simulink model "Lab2"  (R2024b)
settings: Solver=FixedStepAuto  StartTime=0.0  StopTime=10.0  RelTol=1e-3  EnableMultiTasking=on
undefined symbols (not defined in the file): BOOL, DINT, OTL, slplc
libraries: simulink x8, arduinolib x3
(part 1 of 8)
settings Model: ExtModeTrigDuration=2  Creator=CoffeElliot  LastModifiedBy=CoffeElliot
settings SolverCC: AutoInsertRateTranBlk=on
settings OptimizationCC: DefaultParameterBehavior=Inlined  EnhancedBackFolding=on  PassReuseOutputArgsAs=Individual arguments  ZeroExternalMemoryAtStartup=off  ZeroInternalMemoryAtStartup=off  MaxStackSize=64  OptimizeBlockOrder=speed  DifferentSizesBufferReuse=on  OptimizationCustomize=off  EfficientTunableParamExpr=on
settings DebuggingCC: ParameterTunabilityLossMsg=error
settings HardwareCC: ProdBitPerInt=16  ProdBitPerPointer=16  ProdBitPerSizeT=16  ProdBitPerPtrDiffT=16  ProdLargestAtomicFloat=None  ProdWordSize=8  ProdHWDeviceType=Atmel->AVR
settings SFSimCC: MATLABDynamicMemAlloc=off
settings RTWCC: Description=Embedded Coder  SystemTargetFile=ert.tlc  HardwareBoard=Arduino Uno  TemplateMakefile=ert_default_tmf  Toolchain=Arduino AVR  BuildConfiguration=Faster Runs
settings CodeAppCC: ForceParamTrailComments=on  IgnoreCustomStorageClasses=off  OperatorAnnotations=on  SimulinkDataObjDesc=on  SFDataObjDesc=on  InsertBlockDesc=on
settings ERTTargetCC: SupportContinuousTime=on  SupportVariableSizeSignals=on  ExtModeTransport=3  ExtModeStaticAlloc=on  ExtModeAutomaticAllocSize=off  ExtModeStaticAllocSize=250  ExtModeMexFile=ext_xcp  ExtModeIntrfLevel=Level2 - Open

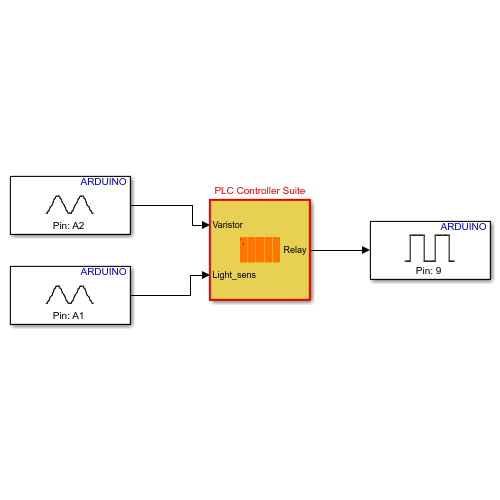
[thumbnail: Simulink's stored preview of the top-level diagram]
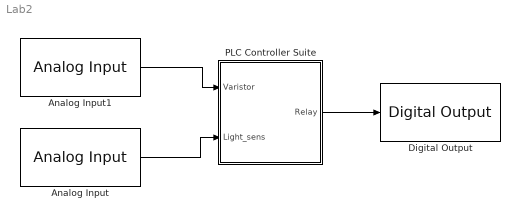
== system Lab2 ==
  Analog Input : arduinolib/Analog Input  pinNumber=1  ReadResultsOnly=off  ConversionTriggerSource=Software  ExternalTriggerType=uint32( 0 )  OutputDataType=uint16  EnableConversionCompleteNotify=off  EnableOuputStatus=off  SampleTime=-1  blockPlatform=arduino
  Analog Input1 : arduinolib/Analog Input  pinNumber=2  ReadResultsOnly=off  ConversionTriggerSource=Software  ExternalTriggerType=uint32( 0 )  OutputDataType=uint16  EnableConversionCompleteNotify=off  EnableOuputStatus=off  SampleTime=-1  blockPlatform=arduino
  Digital Output : arduinolib/Digital Output  pinNumber=9  Direction=output  blockPlatform=arduino
  PLC Controller Suite : Subsystem  TreatAsAtomicUnit=on  mask{PLCBlockType=PLCController, PLCPOUType=PLC Controller}
      mask init:
      | slplc.callbacks.initController(gcb);
      settings: OpenFcn=slplc.callbacks.openPOUBlock(gcb);
      mask Help: web([docroot '/plccoder/ref/plccontrollersuite' '.html']);
      mask DialogControl PLCBlockTitle Prompt: PLC Controller Block
  wires:
  PLC Controller Suite/1(Relay) -> Digital Output/1
  Analog Input1/1 -> PLC Controller Suite/1(Varistor)
  Analog Input/1 -> PLC Controller Suite/2(Light_sens)

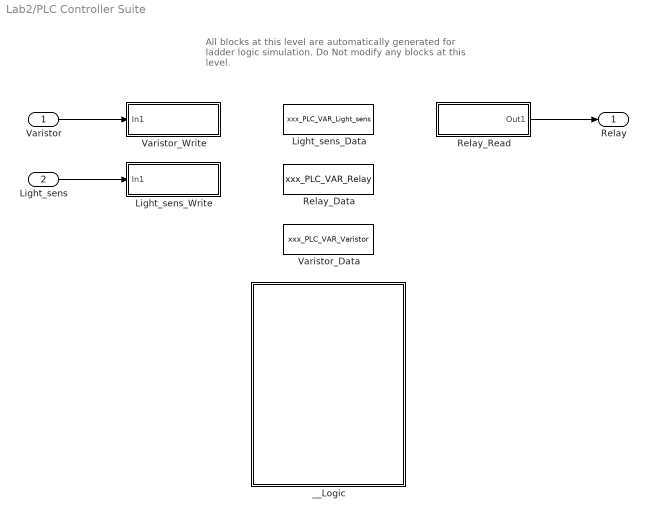
== system Lab2/PLC Controller Suite ==
  note: All blocks at this level are automatically generated for ladder logic simulation.
      | Do Not modify any blocks at this level.
  Varistor : Inport  OutDataTypeStr=double
  Light_sens : Inport  Port=2  OutDataTypeStr=double
  Light_sens_Data : DataStoreMemory  Tag=POUVariable  Priority=10  DataStoreName=xxx_PLC_VAR_Light_sens  InitialValue=1  ShowAdditionalParam=off  OutDataTypeStr=double  Dimensions=1
  Light_sens_Write : Subsystem  Priority=11  DisableCoverage=on  TreatAsAtomicUnit=on  mask{PLCOperandTag=Light_sens, PLCOperandExpression=xxx_PLC_VAR_Light_sens, PLCBlockType=VarWrite, PLCPOUType=VarWrite}
      mask prompts: PLCOperandTag "Operand Tag:"
      mask init:
      | slplc.callbacks.initInstruction(gcb);
      mask Help: web([docroot '/plccoder/ref/varwrite' '.html']);
      mask DialogControl PLCBlockTitle Prompt: Variable Write
      mask Display: disp(get_param(gcb, 'PLCOperandTag'));
  Relay_Data : DataStoreMemory  Tag=POUVariable  Priority=10  DataStoreName=xxx_PLC_VAR_Relay  ShowAdditionalParam=off  OutDataTypeStr=boolean  Dimensions=1
  Relay_Read : Subsystem  Priority=13  DisableCoverage=on  TreatAsAtomicUnit=on  mask{PLCOperandTag=Relay, PLCOperandExpression=xxx_PLC_VAR_Relay, PLCBlockType=VarRead, PLCPOUType=VarRead}
      mask prompts: PLCOperandTag "Operand Tag"
      mask init:
      | block = gcb;
      | maskObj = Simulink.Mask.get(block);
      | maskObj.Display = sprintf('disp(''%s'');', PLCOperandTag);
      | slplc.callbacks.initInstruction(gcb);
      mask Help: web([docroot '/plccoder/ref/varread' '.html']);
      mask DialogControl PLCBlockTitle Prompt: Variable Read
      mask Display: disp('Relay');
  Varistor_Data : DataStoreMemory  Tag=POUVariable  Priority=10  DataStoreName=xxx_PLC_VAR_Varistor  InitialValue=1  ShowAdditionalParam=off  OutDataTypeStr=double  Dimensions=1
  Varistor_Write : Subsystem  Priority=11  DisableCoverage=on  TreatAsAtomicUnit=on  mask{PLCOperandTag=Varistor, PLCOperandExpression=xxx_PLC_VAR_Varistor, PLCBlockType=VarWrite, PLCPOUType=VarWrite}
      mask prompts: PLCOperandTag "Operand Tag:"
      mask init:
      | slplc.callbacks.initInstruction(gcb);
      mask Help: web([docroot '/plccoder/ref/varwrite' '.html']);
      mask DialogControl PLCBlockTitle Prompt: Variable Write
      mask Display: disp(get_param(gcb, 'PLCOperandTag'));
  __Logic : Subsystem  Priority=12  TreatAsAtomicUnit=on
  Relay : Outport
  wires:
  Varistor/1 -> Varistor_Write/1(In1)
  Relay_Read/1(Out1) -> Relay/1
  Light_sens/1 -> Light_sens_Write/1(In1)

== system Lab2/PLC Controller Suite/Light_sens_Write ==
  In1 : Inport
  __CoreVarWrite : Subsystem  Tag=CoreVarWriteBlock  DisableCoverage=on  TreatAsAtomicUnit=on  mask{PLCBlockType=CoreVarWrite}
      mask init:
      | slplc.callbacks.initCoreVariable(gcb, 'write');
      mask DialogControl PLCBlockTitle Prompt: Core Variable Write
  wires:
  In1/1 -> __CoreVarWrite/1(u)

== system Lab2/PLC Controller Suite/Relay_Read ==
  __CoreVarRead : Subsystem  Tag=CoreVarReadBlock  DisableCoverage=on  TreatAsAtomicUnit=on  mask{PLCBlockType=CoreVarRead}
      mask init:
      | slplc.callbacks.initCoreVariable(gcb, 'read');
      mask DialogControl PLCBlockTitle Prompt: Core Variable Read
  Out1 : Outport  VectorParamsAs1DForOutWhenUnconnected=off
  wires:
  __CoreVarRead/1(y) -> Out1/1

== system Lab2/PLC Controller Suite/Varistor_Write ==
  In1 : Inport
  __CoreVarWrite : Subsystem  Tag=CoreVarWriteBlock  DisableCoverage=on  TreatAsAtomicUnit=on  mask{PLCBlockType=CoreVarWrite}
      mask init:
      | slplc.callbacks.initCoreVariable(gcb, 'write');
      mask DialogControl PLCBlockTitle Prompt: Core Variable Write
  wires:
  In1/1 -> __CoreVarWrite/1(u)

== system Lab2/PLC Controller Suite/__Logic ==
  Controller Tags : Subsystem  Tag=ControllerVariableSS  DisableCoverage=on  TreatAsAtomicUnit=on  mask{PLCVarVaristorName=Varistor, PLCVarVaristorAddress=<empty>, PLCVarVaristorMapping=Input Symbol, PLCVarVaristorPortIndex=1, PLCVarVaristorDataType=double, PLCVarVaristorSize=1, PLCVarVaristorInitialValue=1, PLCVarVaristorToDelete=off, PLCVarLight_sensName=Light_sens, PLCVarLight_sensAddress=<empty>, PLCVarLight_sensMapping=Input Symbol, PLCVarLight_sensPortIndex=2, PLCVarLight_sensDataType=double, PLCVarLight_sensSize=1, PLCVarLight_sensInitialValue=1, PLCVarLight_sensToDelete=off, PLCVarRelayName=Relay, PLCVarRelayAddress=<empty>, PLCVarRelayMapping=Output Symbol, PLCVarRelayPortIndex=1, PLCVarRelayDataType=boolean, PLCVarRelaySize=1, PLCVarRelayInitialValue=0, PLCVarRelayToDelete=off}
      mask init:
      | slplc.callbacks.initControllerVarSS(gcb);
      settings: OpenFcn=slplc.callbacks.openControllerVariableSS(gcb);
      mask Help: web([docroot '/plccoder/ref/controllertags' '.html']);
      mask TypeOptions PLCVarVaristorMapping: Global Variable | Input Symbol | Output Symbol
      mask TypeOptions PLCVarVaristorPortIndex: 1 | 2 | 3
      mask TypeOptions PLCVarLight_sensMapping: Global Variable | Input Symbol | Output Symbol
      mask TypeOptions PLCVarLight_sensPortIndex: 1 | 2 | 3
      mask TypeOptions PLCVarRelayMapping: Global Variable | Input Symbol | Output Symbol
      mask TypeOptions PLCVarRelayPortIndex: 1 | 2 | 3
      mask DialogControl PLCBlockTitle Prompt: Global Variable and Symbol Spreadsheet
      mask DialogControl PLCVarListHeaderName Prompt: Name
      mask DialogControl PLCVarListHeaderAddress Prompt: Address (At)
      mask DialogControl PLCVarListHeaderMapping Prompt: Mapping Type
      mask DialogControl PLCVarListHeaderPortIndex Prompt: Port
      mask DialogControl PLCVarListHeaderDataType Prompt: Data Type
      mask DialogControl PLCVarListHeaderSize Prompt: Size
      mask DialogControl PLCVarListHeaderInitialValue Prompt: Initial Value
      mask DialogControl PLCVarListHeaderToDelete Prompt: Delete
  Task : Subsystem  TreatAsAtomicUnit=on  mask{PLCBlockType=Task, PLCPOUType=Task, PLCTaskWatchDog=0}
      settings: OpenFcn=slplc.callbacks.openTaskBlock(gcb);
      mask Help: web([docroot '/plccoder/ref/task' '.html']);
      mask DialogControl PLCBlockTitle Prompt: Task
  Up to Parent POU : Subsystem  DisableCoverage=on  TreatAsAtomicUnit=on  mask{PLCBlockType=OpenParentPOU}
      settings: OpenFcn=slplc.callbacks.openParentPOUBlock(gcb);
      mask Help: web([docroot '/plccoder/ref/uptoparentpou' '.html']);
      mask DialogControl PLCBlockTitle Prompt: Add Single Rung

== system Lab2/PLC Controller Suite/Light_sens_Write/__CoreVarWrite ==
  u : Inport
  DataWrite : DataStoreWrite  DataStoreName=xxx_PLC_VAR_Light_sens  IndexOptions=Index vector (dialog)  Indices=1  OutputSizes=1
  wires:
  u/1 -> DataWrite/1

== system Lab2/PLC Controller Suite/Relay_Read/__CoreVarRead ==
  DataRead : DataStoreRead  DataStoreName=xxx_PLC_VAR_Relay  IndexOptions=Index vector (dialog)  Indices=1  OutputSizes=1
  y : Outport  VectorParamsAs1DForOutWhenUnconnected=off
  wires:
  DataRead/1 -> y/1

== system Lab2/PLC Controller Suite/Varistor_Write/__CoreVarWrite ==
  u : Inport
  DataWrite : DataStoreWrite  DataStoreName=xxx_PLC_VAR_Varistor  IndexOptions=Index vector (dialog)  Indices=1  OutputSizes=1
  wires:
  u/1 -> DataWrite/1

== system Lab2/PLC Controller Suite/__Logic/Controller Tags ==

== system Lab2/PLC Controller Suite/__Logic/Task ==
  Program : Subsystem  TreatAsAtomicUnit=on  mask{PLCPOUType=Program, PLCPOULanguage=LD, PLCBlockType=LDProgram}
      mask prompts: PLCPOUType "POU Type:"
      mask init:
      | slplc.callbacks.initProgram(gcb);
      settings: OpenFcn=slplc.callbacks.openPOUBlock(gcb);
      mask Help: web([docroot '/plccoder/ref/ldprogram' '.html']);
      mask DialogControl PLCBlockTitle Prompt: Program
      mask DialogControl PLCEditPOU Prompt: Edit POU
      mask DialogControl PLCEditInterface Prompt: Edit Variables
  Up to Parent POU : Subsystem  DisableCoverage=on  TreatAsAtomicUnit=on  mask{PLCBlockType=OpenParentPOU}
      settings: OpenFcn=slplc.callbacks.openParentPOUBlock(gcb);
      mask Help: web([docroot '/plccoder/ref/uptoparentpou' '.html']);
      mask DialogControl PLCBlockTitle Prompt: Add Single Rung

== system Lab2/PLC Controller Suite/__Logic/Up to Parent POU ==

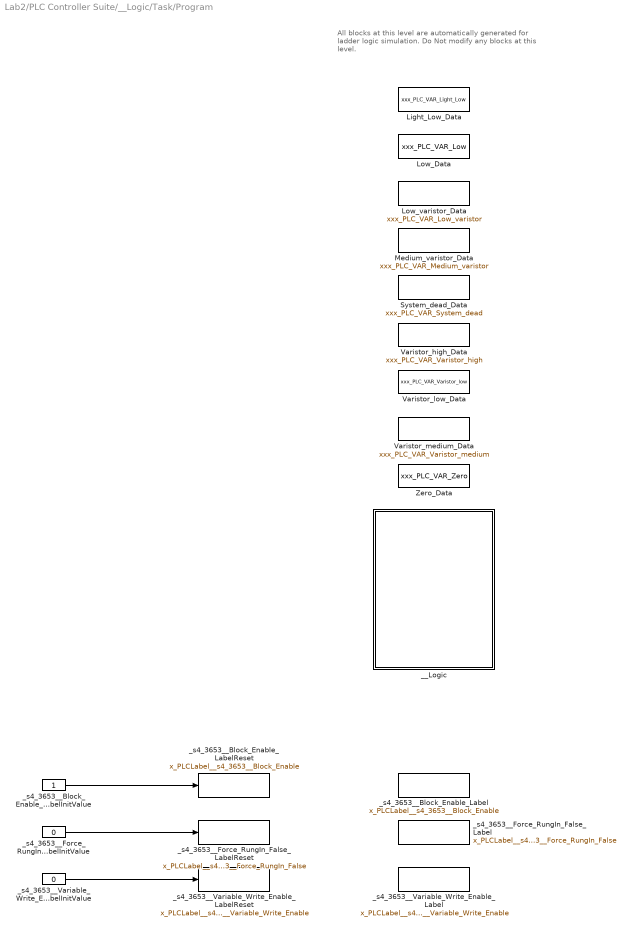
== system Lab2/PLC Controller Suite/__Logic/Task/Program ==
  note: All blocks at this level are automatically generated for ladder logic simulation.
      | Do Not modify any blocks at this level.
  Light_Low_Data : DataStoreMemory  Tag=POUVariable  Priority=10  DataStoreName=xxx_PLC_VAR_Light_Low  InitialValue=false  ShowAdditionalParam=off  OutDataTypeStr=BOOL  Dimensions=1
  Low_Data : DataStoreMemory  Tag=POUVariable  Priority=10  DataStoreName=xxx_PLC_VAR_Low  InitialValue=1000  ShowAdditionalParam=off  OutDataTypeStr=double  Dimensions=1
  Low_varistor_Data : DataStoreMemory  Tag=POUVariable  Priority=10  DataStoreName=xxx_PLC_VAR_Low_varistor  InitialValue=1000  ShowAdditionalParam=off  OutDataTypeStr=double  Dimensions=1
  Medium_varistor_Data : DataStoreMemory  Tag=POUVariable  Priority=10  DataStoreName=xxx_PLC_VAR_Medium_varistor  InitialValue=2500  ShowAdditionalParam=off  OutDataTypeStr=double  Dimensions=1
  System_dead_Data : DataStoreMemory  Tag=POUVariable  Priority=10  DataStoreName=xxx_PLC_VAR_System_dead  InitialValue=false  ShowAdditionalParam=off  OutDataTypeStr=BOOL  Dimensions=1
  Varistor_high_Data : DataStoreMemory  Tag=POUVariable  Priority=10  DataStoreName=xxx_PLC_VAR_Varistor_high  InitialValue=false  ShowAdditionalParam=off  OutDataTypeStr=BOOL  Dimensions=1
  Varistor_low_Data : DataStoreMemory  Tag=POUVariable  Priority=10  DataStoreName=xxx_PLC_VAR_Varistor_low  InitialValue=false  ShowAdditionalParam=off  OutDataTypeStr=BOOL  Dimensions=1
  Varistor_medium_Data : DataStoreMemory  Tag=POUVariable  Priority=10  DataStoreName=xxx_PLC_VAR_Varistor_medium  InitialValue=false  ShowAdditionalParam=off  OutDataTypeStr=BOOL  Dimensions=1
  Zero_Data : DataStoreMemory  Tag=POUVariable  Priority=10  DataStoreName=xxx_PLC_VAR_Zero  InitialValue=10  ShowAdditionalParam=off  OutDataTypeStr=double  Dimensions=1
  __Logic : Subsystem  Priority=12  TreatAsAtomicUnit=on
  _s4_3653__Block_Enable_Label : DataStoreMemory  Priority=10  DataStoreName=x_PLCLabel__s4_3653__Block_Enable  InitialValue=1  ShowAdditionalParam=off  OutDataTypeStr=BOOL  Dimensions=1
  _s4_3653__Block_Enable_LabelInitValue : Constant  OutDataTypeStr=BOOL
  _s4_3653__Block_Enable_LabelReset : DataStoreWrite  Priority=11  DataStoreName=x_PLCLabel__s4_3653__Block_Enable  IndexOptions=Index vector (dialog)  Indices=1  OutputSizes=1
  _s4_3653__Force_RungIn_False_Label : DataStoreMemory  Priority=10  DataStoreName=x_PLCLabel__s4_3653__Force_RungIn_False  ShowAdditionalParam=off  OutDataTypeStr=BOOL  Dimensions=1
  _s4_3653__Force_RungIn_False_LabelInitValue : Constant  Value=0  OutDataTypeStr=BOOL
  _s4_3653__Force_RungIn_False_LabelReset : DataStoreWrite  Priority=11  DataStoreName=x_PLCLabel__s4_3653__Force_RungIn_False  IndexOptions=Index vector (dialog)  Indices=1  OutputSizes=1
  _s4_3653__Variable_Write_Enable_Label : DataStoreMemory  Priority=10  DataStoreName=x_PLCLabel__s4_3653__Variable_Write_Enable  ShowAdditionalParam=off  OutDataTypeStr=BOOL  Dimensions=1
  _s4_3653__Variable_Write_Enable_LabelInitValue : Constant  Value=0  OutDataTypeStr=BOOL
  _s4_3653__Variable_Write_Enable_LabelReset : DataStoreWrite  Priority=11  DataStoreName=x_PLCLabel__s4_3653__Variable_Write_Enable  IndexOptions=Index vector (dialog)  Indices=1  OutputSizes=1
  wires:
  _s4_3653__Block_Enable_LabelInitValue/1 -> _s4_3653__Block_Enable_LabelReset/1
  _s4_3653__Variable_Write_Enable_LabelInitValue/1 -> _s4_3653__Variable_Write_Enable_LabelReset/1
  _s4_3653__Force_RungIn_False_LabelInitValue/1 -> _s4_3653__Force_RungIn_False_LabelReset/1

== system Lab2/PLC Controller Suite/__Logic/Task/Up to Parent POU ==

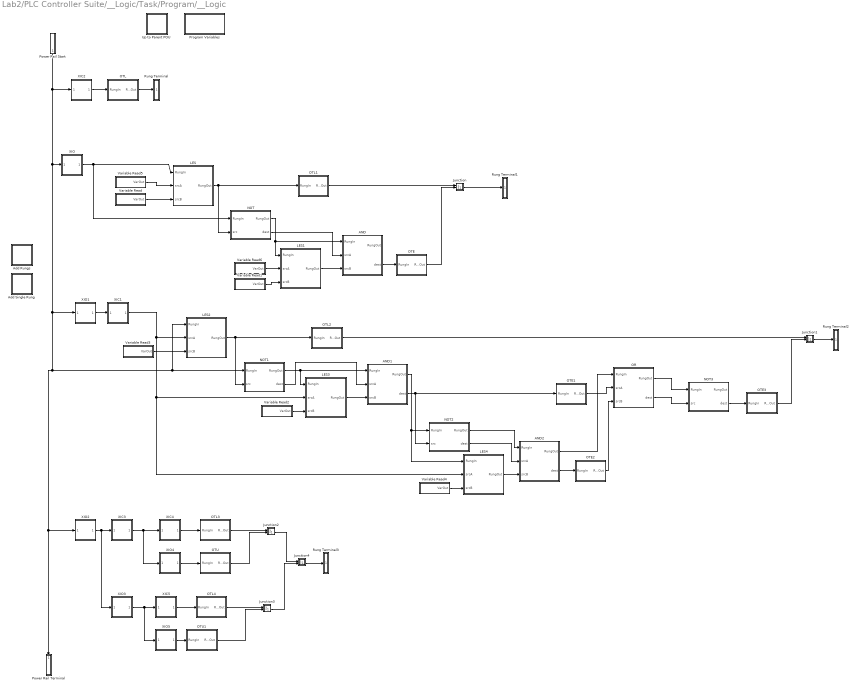
== system Lab2/PLC Controller Suite/__Logic/Task/Program/__Logic ==
  AND : Subsystem  Priority=1  TreatAsAtomicUnit=on  mask{PLCBlockType=AND, PLCPOUType=stdFC}
      mask Help: web([docroot '/plccoder/ref/and' '.html']);
      mask DialogControl PLCBlockTitle Prompt: Bitwise And (AND)
      mask DialogControl PLCBlockDesc Prompt: Perform a bitwise AND operation using the bits in Source A and Source B and place the result in Destination.
      mask Display: disp('AND');
  AND1 : Subsystem  Priority=1  TreatAsAtomicUnit=on  mask{PLCBlockType=AND, PLCPOUType=stdFC}
      mask Help: web([docroot '/plccoder/ref/and' '.html']);
      mask DialogControl PLCBlockTitle Prompt: Bitwise And (AND)
      mask DialogControl PLCBlockDesc Prompt: Perform a bitwise AND operation using the bits in Source A and Source B and place the result in Destination.
      mask Display: disp('AND');
  AND2 : Subsystem  Priority=1  TreatAsAtomicUnit=on  mask{PLCBlockType=AND, PLCPOUType=stdFC}
      mask Help: web([docroot '/plccoder/ref/and' '.html']);
      mask DialogControl PLCBlockTitle Prompt: Bitwise And (AND)
      mask DialogControl PLCBlockDesc Prompt: Perform a bitwise AND operation using the bits in Source A and Source B and place the result in Destination.
      mask Display: disp('AND');
  Add Rungs : Subsystem  DisableCoverage=on  TreatAsAtomicUnit=on  mask{PLCRungNumberToAdd=2, PLCBlockType=AddRungs}
      mask prompts: PLCRungNumberToAdd "Rung Number:"
      mask Help: web([docroot '/plccoder/ref/addrungs' '.html']);
      mask DialogControl PLCAddRungs Prompt: Add Rungs
      mask DialogControl PLCRungAddButton Prompt: Add
      mask DialogControl PLCRungAddButton Callback: slplc.callbacks.addLadderRungs(gcb);
      mask Display: disp(sprintf(['Add' newline 'Rungs']));
  Add Single Rung : Subsystem  DisableCoverage=on  TreatAsAtomicUnit=on  mask{PLCRungNumberToAdd=1, PLCBlockType=AddSingleRung}
      settings: OpenFcn=slplc.callbacks.addLadderRungs(gcb);
      mask Help: web([docroot '/plccoder/ref/addsinglerung' '.html']);
      mask DialogControl PLCAddRung Prompt: Add Single Rung
      mask Display: disp(sprintf(['Add' newline '1 Rung']));
  Junction : Subsystem  DisableCoverage=on  TreatAsAtomicUnit=on  mask{PLCBlockType=Junction, PLCPOUType=BranchJunction}
      mask Help: web([docroot '/plccoder/ref/junction' '.html']);
      mask DialogControl PLCBlockTitle Prompt: Rung Merge Point
      mask DialogControl PLCBlockDesc Prompt: This is the ladder diagram rung merge point.
  Junction1 : Subsystem  DisableCoverage=on  TreatAsAtomicUnit=on  mask{PLCBlockType=Junction, PLCPOUType=BranchJunction}
      mask Help: web([docroot '/plccoder/ref/junction' '.html']);
      mask DialogControl PLCBlockTitle Prompt: Rung Merge Point
      mask DialogControl PLCBlockDesc Prompt: This is the ladder diagram rung merge point.
  Junction2 : Subsystem  DisableCoverage=on  TreatAsAtomicUnit=on  mask{PLCBlockType=Junction, PLCPOUType=BranchJunction}
      mask Help: web([docroot '/plccoder/ref/junction' '.html']);
      mask DialogControl PLCBlockTitle Prompt: Rung Merge Point
      mask DialogControl PLCBlockDesc Prompt: This is the ladder diagram rung merge point.
  Junction3 : Subsystem  DisableCoverage=on  TreatAsAtomicUnit=on  mask{PLCBlockType=Junction, PLCPOUType=BranchJunction}
      mask Help: web([docroot '/plccoder/ref/junction' '.html']);
      mask DialogControl PLCBlockTitle Prompt: Rung Merge Point
      mask DialogControl PLCBlockDesc Prompt: This is the ladder diagram rung merge point.
  Junction4 : Subsystem  DisableCoverage=on  TreatAsAtomicUnit=on  mask{PLCBlockType=Junction, PLCPOUType=BranchJunction}
      mask Help: web([docroot '/plccoder/ref/junction' '.html']);
      mask DialogControl PLCBlockTitle Prompt: Rung Merge Point
      mask DialogControl PLCBlockDesc Prompt: This is the ladder diagram rung merge point.
  LES : Subsystem  Priority=8  TreatAsAtomicUnit=on  mask{PLCBlockType=LES, PLCPOUType=stdFC}
      mask Help: web([docroot '/plccoder/ref/les' '.html']);
      mask DialogControl PLCBlockTitle Prompt: Less Than (LES)
      mask DialogControl PLCBlockDesc Prompt: Test whether Source A is less than Source B.
      mask Display: disp('LES');
  LES1 : Subsystem  Priority=1  TreatAsAtomicUnit=on  mask{PLCBlockType=LES, PLCPOUType=stdFC}
      mask Help: web([docroot '/plccoder/ref/les' '.html']);
      mask DialogControl PLCBlockTitle Prompt: Less Than (LES)
      mask DialogControl PLCBlockDesc Prompt: Test whether Source A is less than Source B.
      mask Display: disp('LES');
  LES2 : Subsystem  Priority=1  TreatAsAtomicUnit=on  mask{PLCBlockType=LES, PLCPOUType=stdFC}
      mask Help: web([docroot '/plccoder/ref/les' '.html']);
      mask DialogControl PLCBlockTitle Prompt: Less Than (LES)
      mask DialogControl PLCBlockDesc Prompt: Test whether Source A is less than Source B.
      mask Display: disp('LES');
  LES3 : Subsystem  Priority=1  TreatAsAtomicUnit=on  mask{PLCBlockType=LES, PLCPOUType=stdFC}
      mask Help: web([docroot '/plccoder/ref/les' '.html']);
      mask DialogControl PLCBlockTitle Prompt: Less Than (LES)
      mask DialogControl PLCBlockDesc Prompt: Test whether Source A is less than Source B.
      mask Display: disp('LES');
  LES4 : Subsystem  Priority=1  TreatAsAtomicUnit=on  mask{PLCBlockType=LES, PLCPOUType=stdFC}
      mask Help: web([docroot '/plccoder/ref/les' '.html']);
      mask DialogControl PLCBlockTitle Prompt: Less Than (LES)
      mask DialogControl PLCBlockDesc Prompt: Test whether Source A is less than Source B.
      mask Display: disp('LES');
  NOT : Subsystem  Priority=1  TreatAsAtomicUnit=on  mask{PLCBlockType=NOT, PLCPOUType=stdFC}
      mask Help: web([docroot '/plccoder/ref/not' '.html']);
      mask DialogControl PLCBlockTitle Prompt: Bitwise Not (NOT)
      mask DialogControl PLCBlockDesc Prompt: Perform a bitwise inversion of the Source and place the result in Destination.
      mask Display: disp('NOT');
  NOT1 : Subsystem  Priority=1  TreatAsAtomicUnit=on  mask{PLCBlockType=NOT, PLCPOUType=stdFC}
      mask Help: web([docroot '/plccoder/ref/not' '.html']);
      mask DialogControl PLCBlockTitle Prompt: Bitwise Not (NOT)
      mask DialogControl PLCBlockDesc Prompt: Perform a bitwise inversion of the Source and place the result in Destination.
      mask Display: disp('NOT');
  NOT2 : Subsystem  Priority=1  TreatAsAtomicUnit=on  mask{PLCBlockType=NOT, PLCPOUType=stdFC}
      mask Help: web([docroot '/plccoder/ref/not' '.html']);
      mask DialogControl PLCBlockTitle Prompt: Bitwise Not (NOT)
      mask DialogControl PLCBlockDesc Prompt: Perform a bitwise inversion of the Source and place the result in Destination.
      mask Display: disp('NOT');
  NOT3 : Subsystem  Priority=1  TreatAsAtomicUnit=on  mask{PLCBlockType=NOT, PLCPOUType=stdFC}
      mask Help: web([docroot '/plccoder/ref/not' '.html']);
      mask DialogControl PLCBlockTitle Prompt: Bitwise Not (NOT)
      mask DialogControl PLCBlockDesc Prompt: Perform a bitwise inversion of the Source and place the result in Destination.
      mask Display: disp('NOT');
  OR : Subsystem  Priority=1  TreatAsAtomicUnit=on  mask{PLCBlockType=OR, PLCPOUType=stdFC}
      mask Help: web([docroot '/plccoder/ref/or' '.html']);
      mask DialogControl PLCBlockTitle Prompt: Bitwise Or
      mask DialogControl PLCBlockDesc Prompt: Perform a bitwise OR operation using the bits in Source A and Source B and place the result in Destination.
      mask Display: disp('OR');
  OTE : Subsystem  Priority=3  TreatAsAtomicUnit=on  mask{PLCOperandTag=Light_Low, PLCBlockType=OTE, PLCPOUType=Coil, PLCOperandExpression=xxx_PLC_VAR_Light_Low}
      mask prompts: PLCOperandTag "Operand Tag:"
      mask init:
      | slplc.callbacks.initInstruction(gcb);
      settings: AttributesFormatString=%<PLCOperandTag>
      mask Help: web([docroot '/plccoder/ref/ote' '.html']);
      mask DialogControl PLCBlockTitle Prompt: Output Energize (OTE)
  OTE1 : Subsystem  Priority=3  TreatAsAtomicUnit=on  mask{PLCOperandTag=Varistor_low, PLCBlockType=OTE, PLCPOUType=Coil, PLCOperandExpression=xxx_PLC_VAR_Varistor_low}
      mask prompts: PLCOperandTag "Operand Tag:"
      mask init:
      | slplc.callbacks.initInstruction(gcb);
      settings: AttributesFormatString=%<PLCOperandTag>
      mask Help: web([docroot '/plccoder/ref/ote' '.html']);
      mask DialogControl PLCBlockTitle Prompt: Output Energize (OTE)
  OTE2 : Subsystem  Priority=3  TreatAsAtomicUnit=on  mask{PLCOperandTag=Varistor_medium, PLCBlockType=OTE, PLCPOUType=Coil, PLCOperandExpression=xxx_PLC_VAR_Varistor_medium}
      mask prompts: PLCOperandTag "Operand Tag:"
      mask init:
      | slplc.callbacks.initInstruction(gcb);
      settings: AttributesFormatString=%<PLCOperandTag>
      mask Help: web([docroot '/plccoder/ref/ote' '.html']);
      mask DialogControl PLCBlockTitle Prompt: Output Energize (OTE)
  OTE3 : Subsystem  Priority=3  TreatAsAtomicUnit=on  mask{PLCOperandTag=Varistor_high, PLCBlockType=OTE, PLCPOUType=Coil, PLCOperandExpression=xxx_PLC_VAR_Varistor_high}
      mask prompts: PLCOperandTag "Operand Tag:"
      mask init:
      | slplc.callbacks.initInstruction(gcb);
      settings: AttributesFormatString=%<PLCOperandTag>
      mask Help: web([docroot '/plccoder/ref/ote' '.html']);
      mask DialogControl PLCBlockTitle Prompt: Output Energize (OTE)
  OTL : Subsystem  Priority=3  TreatAsAtomicUnit=on  mask{PLCOperandTag=Relay, PLCBlockType=OTL, PLCPOUType=Coil, PLCOperandExpression=xxx_PLC_VAR_Relay}
      mask prompts: PLCOperandTag "Operand Tag:"
      mask init:
      | slplc.callbacks.initInstruction(gcb);
      settings: AttributesFormatString=%<PLCOperandTag>
      mask Help: web([docroot '/plccoder/ref/otl' '.html']);
      mask DialogControl PLCBlockTitle Prompt: Output Latch (OTL)
      mask Display: disp('L');
  OTL1 : Subsystem  Priority=9  TreatAsAtomicUnit=on  mask{PLCOperandTag=System_dead, PLCBlockType=OTL, PLCPOUType=Coil, PLCOperandExpression=xxx_PLC_VAR_System_dead}
      mask prompts: PLCOperandTag "Operand Tag:"
      mask init:
      | slplc.callbacks.initInstruction(gcb);
      settings: AttributesFormatString=%<PLCOperandTag>
      mask Help: web([docroot '/plccoder/ref/otl' '.html']);
      mask DialogControl PLCBlockTitle Prompt: Output Latch (OTL)
      mask Display: disp('L');
  OTL2 : Subsystem  Priority=3  TreatAsAtomicUnit=on  mask{PLCOperandTag=Relay, PLCBlockType=OTL, PLCPOUType=Coil, PLCOperandExpression=xxx_PLC_VAR_Relay}
      mask prompts: PLCOperandTag "Operand Tag:"
      mask init:
      | slplc.callbacks.initInstruction(gcb);
      settings: AttributesFormatString=%<PLCOperandTag>
      mask Help: web([docroot '/plccoder/ref/otl' '.html']);
      mask DialogControl PLCBlockTitle Prompt: Output Latch (OTL)
      mask Display: disp('L');
  OTL3 : Subsystem  Priority=3  TreatAsAtomicUnit=on  mask{PLCOperandTag=System_dead, PLCBlockType=OTL, PLCPOUType=Coil, PLCOperandExpression=xxx_PLC_VAR_System_dead}
      mask prompts: PLCOperandTag "Operand Tag:"
      mask init:
      | slplc.callbacks.initInstruction(gcb);
      settings: AttributesFormatString=%<PLCOperandTag>
      mask Help: web([docroot '/plccoder/ref/otl' '.html']);
      mask DialogControl PLCBlockTitle Prompt: Output Latch (OTL)
      mask Display: disp('L');
  OTL4 : Subsystem  Priority=3  TreatAsAtomicUnit=on  mask{PLCOperandTag=Relay, PLCBlockType=OTL, PLCPOUType=Coil, PLCOperandExpression=xxx_PLC_VAR_Relay}
      mask prompts: PLCOperandTag "Operand Tag:"
      mask init:
      | slplc.callbacks.initInstruction(gcb);
      settings: AttributesFormatString=%<PLCOperandTag>
      mask Help: web([docroot '/plccoder/ref/otl' '.html']);
      mask DialogControl PLCBlockTitle Prompt: Output Latch (OTL)
      mask Display: disp('L');
  OTU : Subsystem  Priority=4  TreatAsAtomicUnit=on  mask{PLCOperandTag=Relay, PLCBlockType=OTU, PLCPOUType=Coil, PLCOperandExpression=xxx_PLC_VAR_Relay}
      mask prompts: PLCOperandTag "Operand Tag:"
      mask init:
      | slplc.callbacks.initInstruction(gcb);
      settings: AttributesFormatString=%<PLCOperandTag>
      mask Help: web([docroot '/plccoder/ref/otu' '.html']);
      mask DialogControl PLCBlockTitle Prompt: Output Unlatch (OTU)
      mask Display: disp('U');
  OTU1 : Subsystem  Priority=4  TreatAsAtomicUnit=on  mask{PLCOperandTag=Relay, PLCBlockType=OTU, PLCPOUType=Coil, PLCOperandExpression=xxx_PLC_VAR_Relay}
      mask prompts: PLCOperandTag "Operand Tag:"
      mask init:
      | slplc.callbacks.initInstruction(gcb);
      settings: AttributesFormatString=%<PLCOperandTag>
      mask Help: web([docroot '/plccoder/ref/otu' '.html']);
      mask DialogControl PLCBlockTitle Prompt: Output Unlatch (OTU)
      mask Display: disp('U');
  Power Rail Start : Subsystem  Priority=1  DisableCoverage=on  TreatAsAtomicUnit=on  mask{PLCBlockType=PowerRailStart}
      mask Help: web([docroot '/plccoder/ref/powerrailstart' '.html']);
      mask DialogControl PLCBlockTitle Prompt: Power Rail Start
      mask DialogControl PLCBlockDesc Prompt: This is the ladder diagram left power rail start block.
  Power Rail Terminal : Subsystem  DisableCoverage=on  TreatAsAtomicUnit=on  mask{PLCBlockType=PowerRailTerminal}
      mask Help: web([docroot '/plccoder/ref/powerrailterminal' '.html']);
      mask DialogControl PLCBlockTitle Prompt: Power Rail Terminal
      mask DialogControl PLCBlockDesc Prompt: This is the ladder diagram left power rail terminal block.
  Program Variables : Subsystem  Tag=ProgramVariableSS  DisableCoverage=on  TreatAsAtomicUnit=on  mask{PLCVarLight_LowName=Light_Low, PLCVarLight_LowScope=Local, PLCVarLight_LowPortType=Hidden, PLCVarLight_LowPortIndex=12, PLCVarLight_LowDataType=BOOL, PLCVarLight_LowSize=1, PLCVarLight_LowInitialValue=false, PLCVarLight_LowToDelete=off, PLCVarLowName=Low, PLCVarLowScope=Local, PLCVarLowPortType=Hidden, PLCVarLowPortIndex=12, PLCVarLowDataType=double, PLCVarLowSize=1, PLCVarLowInitialValue=1000, PLCVarLowToDelete=off, PLCVarLow_varistorName=Low_varistor, PLCVarLow_varistorScope=Local, PLCVarLow_varistorPortType=Hidden, PLCVarLow_varistorPortIndex=12, PLCVarLow_varistorDataType=double, PLCVarLow_varistorSize=1, PLCVarLow_varistorInitialValue=1000, PLCVarLow_varistorToDelete=off, PLCVarMedium_varistorName=Medium_varistor, PLCVarMedium_varistorScope=Local, PLCVarMedium_varistorPortType=Hidden, PLCVarMedium_varistorPortIndex=12, PLCVarMedium_varistorDataType=double, PLCVarMedium_varistorSize=1, PLCVarMedium_varistorInitialValue=2500, PLCVarMedium_varistorToDelete=off, PLCVarSystem_deadName=System_dead, PLCVarSystem_deadScope=Local, PLCVarSystem_deadPortType=Hidden, PLCVarSystem_deadPortIndex=12, PLCVarSystem_deadDataType=BOOL, PLCVarSystem_deadSize=1, PLCVarSystem_deadInitialValue=false, PLCVarSystem_deadToDelete=off, PLCVarVaristor_highName=Varistor_high, PLCVarVaristor_highScope=Local, PLCVarVaristor_highPortType=Hidden, PLCVarVaristor_highPortIndex=12, PLCVarVaristor_highDataType=BOOL, PLCVarVaristor_highSize=1, PLCVarVaristor_highInitialValue=false, PLCVarVaristor_highToDelete=off, PLCVarVaristor_lowName=Varistor_low, PLCVarVaristor_lowScope=Local, PLCVarVaristor_lowPortType=Hidden, PLCVarVaristor_lowPortIndex=12, PLCVarVaristor_lowDataType=BOOL, PLCVarVaristor_lowSize=1, PLCVarVaristor_lowInitialValue=false, PLCVarVaristor_lowToDelete=off, PLCVarVaristor_mediumName=Varistor_medium, PLCVarVaristor_mediumScope=Local, PLCVarVaristor_mediumPortType=Hidden, PLCVarVaristor_mediumPortIndex=12, PLCVarVaristor_mediumDataType=BOOL, PLCVarVaristor_mediumSize=1, PLCVarVaristor_mediumInitialValue=false, PLCVarVaristor_mediumToDelete=off, PLCVarZeroName=Zero, PLCVarZeroScope=Local, PLCVarZeroPortType=Hidden, PLCVarZeroPortIndex=12, PLCVarZeroDataType=double, PLCVarZeroSize=1, PLCVarZeroInitialValue=10, PLCVarZeroToDelete=off, PLCVarLight_sensName=Light_sens, PLCVarLight_sensScope=External, PLCVarLight_sensPortType=Hidden, PLCVarLight_sensPortIndex=12, PLCVarLight_sensDataType=DINT, PLCVarLight_sensSize=-1, PLCVarLight_sensInitialValue=0, PLCVarLight_sensToDelete=off, PLCVarRelayName=Relay, PLCVarRelayScope=External, PLCVarRelayPortType=Hidden, PLCVarRelayPortIndex=12, PLCVarRelayDataType=DINT, PLCVarRelaySize=-1, PLCVarRelayInitialValue=0, PLCVarRelayToDelete=off, PLCVarVaristorName=Varistor, PLCVarVaristorScope=External, PLCVarVaristorPortType=Hidden, PLCVarVaristorPortIndex=12, PLCVarVaristorDataType=DINT, PLCVarVaristorSize=-1, PLCVarVaristorInitialValue=0, PLCVarVaristorToDelete=off}
      mask init:
      | slplc.callbacks.initPOUVarSS(gcb);
      settings: OpenFcn=slplc.callbacks.openProgramVariableSS(gcb);
      mask Help: web([docroot '/plccoder/ref/programvariables' '.html']);
      mask TypeOptions PLCVarLight_LowScope: Local | External
      mask TypeOptions PLCVarLight_LowPortType: Hidden | Inport | Outport
      mask TypeOptions PLCVarLight_LowPortIndex: 1 | 2 | 3 | 4 | 5 | 6 | 7 | 8 | 9 | 10 | 11 | 12
      mask TypeOptions PLCVarLowScope: Local | External
      mask TypeOptions PLCVarLowPortType: Hidden | Inport | Outport
      mask TypeOptions PLCVarLowPortIndex: 1 | 2 | 3 | 4 | 5 | 6 | 7 | 8 | 9 | 10 | 11 | 12
      mask TypeOptions PLCVarLow_varistorScope: Local | External
      mask TypeOptions PLCVarLow_varistorPortType: Hidden | Inport | Outport
      mask TypeOptions PLCVarLow_varistorPortIndex: 1 | 2 | 3 | 4 | 5 | 6 | 7 | 8 | 9 | 10 | 11 | 12
      mask TypeOptions PLCVarMedium_varistorScope: Local | External
      mask TypeOptions PLCVarMedium_varistorPortType: Hidden | Inport | Outport
      mask TypeOptions PLCVarMedium_varistorPortIndex: 1 | 2 | 3 | 4 | 5 | 6 | 7 | 8 | 9 | 10 | 11 | 12
      mask TypeOptions PLCVarSystem_deadScope: Local | External
      mask TypeOptions PLCVarSystem_deadPortType: Hidden | Inport | Outport
      mask TypeOptions PLCVarSystem_deadPortIndex: 1 | 2 | 3 | 4 | 5 | 6 | 7 | 8 | 9 | 10 | 11 | 12
      mask TypeOptions PLCVarVaristor_highScope: Local | External
      mask TypeOptions PLCVarVaristor_highPortType: Hidden | Inport | Outport
      mask TypeOptions PLCVarVaristor_highPortIndex: 1 | 2 | 3 | 4 | 5 | 6 | 7 | 8 | 9 | 10 | 11 | 12
      mask TypeOptions PLCVarVaristor_lowScope: Local | External
      mask TypeOptions PLCVarVaristor_lowPortType: Hidden | Inport | Outport
      mask TypeOptions PLCVarVaristor_lowPortIndex: 1 | 2 | 3 | 4 | 5 | 6 | 7 | 8 | 9 | 10 | 11 | 12
      mask TypeOptions PLCVarVaristor_mediumScope: Local | External
      mask TypeOptions PLCVarVaristor_mediumPortType: Hidden | Inport | Outport
      mask TypeOptions PLCVarVaristor_mediumPortIndex: 1 | 2 | 3 | 4 | 5 | 6 | 7 | 8 | 9 | 10 | 11 | 12
      mask TypeOptions PLCVarZeroScope: Local | External
      mask TypeOptions PLCVarZeroPortType: Hidden | Inport | Outport
      mask TypeOptions PLCVarZeroPortIndex: 1 | 2 | 3 | 4 | 5 | 6 | 7 | 8 | 9 | 10 | 11 | 12
      mask TypeOptions PLCVarLight_sensScope: Local | External
      mask TypeOptions PLCVarLight_sensPortType: Hidden | Inport | Outport
      mask TypeOptions PLCVarLight_sensPortIndex: 1 | 2 | 3 | 4 | 5 | 6 | 7 | 8 | 9 | 10 | 11 | 12
      mask TypeOptions PLCVarRelayScope: Local | External
      mask TypeOptions PLCVarRelayPortType: Hidden | Inport | Outport
      mask TypeOptions PLCVarRelayPortIndex: 1 | 2 | 3 | 4 | 5 | 6 | 7 | 8 | 9 | 10 | 11 | 12
      mask TypeOptions PLCVarVaristorScope: Local | External
      mask TypeOptions PLCVarVaristorPortType: Hidden | Inport | Outport
      mask TypeOptions PLCVarVaristorPortIndex: 1 | 2 | 3 | 4 | 5 | 6 | 7 | 8 | 9 | 10 | 11 | 12
      mask DialogControl PLCBlockTitle Prompt: Program Variable Spreadsheet
      mask DialogControl PLCVarListHeaderName Prompt: Name
      mask DialogControl PLCVarListHeaderScope Prompt: Scope
      mask DialogControl PLCVarListHeaderDataType Prompt: Data Type
      mask DialogControl PLCVarListHeaderSize Prompt: Size
      mask DialogControl PLCVarListHeaderInitialValue Prompt: Initial Value
      mask DialogControl PLCVarListHeaderToDelete Prompt: Delete
  Rung Terminal : Subsystem  Priority=4  DisableCoverage=on  TreatAsAtomicUnit=on  mask{PLCRungTerminalIndex=1, PLCBlockType=RungTerminal}
      settings: AttributesFormatString=Rung %<PLCRungTerminalIndex>
      mask Help: web([docroot '/plccoder/ref/rungterminal' '.html']);
      mask DialogControl PLCBlockTitle Prompt: Rung Terminal
      mask DialogControl PLCBlockDescText Prompt: This is the ladder diagram rung terminal.
  Rung Terminal1 : Subsystem  DisableCoverage=on  TreatAsAtomicUnit=on  mask{PLCRungTerminalIndex=1, PLCBlockType=RungTerminal}
      settings: AttributesFormatString=Rung %<PLCRungTerminalIndex>
      mask Help: web([docroot '/plccoder/ref/rungterminal' '.html']);
      mask DialogControl PLCBlockTitle Prompt: Rung Terminal
      mask DialogControl PLCBlockDescText Prompt: This is the ladder diagram rung terminal.
  Rung Terminal2 : Subsystem  DisableCoverage=on  TreatAsAtomicUnit=on  mask{PLCRungTerminalIndex=1, PLCBlockType=RungTerminal}
      settings: AttributesFormatString=Rung %<PLCRungTerminalIndex>
      mask Help: web([docroot '/plccoder/ref/rungterminal' '.html']);
      mask DialogControl PLCBlockTitle Prompt: Rung Terminal
      mask DialogControl PLCBlockDescText Prompt: This is the ladder diagram rung terminal.
  Rung Terminal3 : Subsystem  DisableCoverage=on  TreatAsAtomicUnit=on  mask{PLCRungTerminalIndex=1, PLCBlockType=RungTerminal}
      settings: AttributesFormatString=Rung %<PLCRungTerminalIndex>
      mask Help: web([docroot '/plccoder/ref/rungterminal' '.html']);
      mask DialogControl PLCBlockTitle Prompt: Rung Terminal
      mask DialogControl PLCBlockDescText Prompt: This is the ladder diagram rung terminal.
  Up to Parent POU : Subsystem  DisableCoverage=on  TreatAsAtomicUnit=on  mask{PLCBlockType=OpenParentPOU}
      settings: OpenFcn=slplc.callbacks.openParentPOUBlock(gcb);
      mask Help: web([docroot '/plccoder/ref/uptoparentpou' '.html']);
      mask DialogControl PLCBlockTitle Prompt: Add Single Rung
  Variable Read : Subsystem  Priority=7  TreatAsAtomicUnit=on  mask{PLCOperandTag=Zero, PLCBlockType=VariableRead, PLCOperandAccess=Read, PLCPOUType=VariableRead, PLCOperandExpression=xxx_PLC_VAR_Zero}
      mask prompts: PLCOperandTag "Data Tag:"
      mask init:
      | block = gcb;
      | maskObj = Simulink.Mask.get(block);
      | maskObj.Display = sprintf('disp(''%s'');', PLCOperandTag);
      | slplc.callbacks.initInstruction(block);
      mask Help: web([docroot '/plccoder/ref/variableread' '.html']);
      mask DialogControl PLCBlockTitle Prompt: Data Tag Read
      mask Display: disp('Zero');
  Variable Read1 : Subsystem  Priority=1  TreatAsAtomicUnit=on  mask{PLCOperandTag=Low, PLCBlockType=VariableRead, PLCOperandAccess=Read, PLCPOUType=VariableRead, PLCOperandExpression=xxx_PLC_VAR_Low}
      mask prompts: PLCOperandTag "Data Tag:"
      mask init:
      | block = gcb;
      | maskObj = Simulink.Mask.get(block);
      | maskObj.Display = sprintf('disp(''%s'');', PLCOperandTag);
      | slplc.callbacks.initInstruction(block);
      mask Help: web([docroot '/plccoder/ref/variableread' '.html']);
      mask DialogControl PLCBlockTitle Prompt: Data Tag Read
      mask Display: disp('Low');
  Variable Read2 : Subsystem  Priority=1  TreatAsAtomicUnit=on  mask{PLCOperandTag=Low_varistor, PLCBlockType=VariableRead, PLCOperandAccess=Read, PLCPOUType=VariableRead, PLCOperandExpression=xxx_PLC_VAR_Low_varistor}
      mask prompts: PLCOperandTag "Data Tag:"
      mask init:
      | block = gcb;
      | maskObj = Simulink.Mask.get(block);
      | maskObj.Display = sprintf('disp(''%s'');', PLCOperandTag);
      | slplc.callbacks.initInstruction(block);
      mask Help: web([docroot '/plccoder/ref/variableread' '.html']);
      mask DialogControl PLCBlockTitle Prompt: Data Tag Read
      mask Display: disp('Low_varistor');
  Variable Read3 : Subsystem  Priority=1  TreatAsAtomicUnit=on  mask{PLCOperandTag=Zero, PLCBlockType=VariableRead, PLCOperandAccess=Read, PLCPOUType=VariableRead, PLCOperandExpression=xxx_PLC_VAR_Zero}
      mask prompts: PLCOperandTag "Data Tag:"
      mask init:
      | block = gcb;
      | maskObj = Simulink.Mask.get(block);
      | maskObj.Display = sprintf('disp(''%s'');', PLCOperandTag);
      | slplc.callbacks.initInstruction(block);
      mask Help: web([docroot '/plccoder/ref/variableread' '.html']);
      mask DialogControl PLCBlockTitle Prompt: Data Tag Read
      mask Display: disp('Zero');
  Variable Read4 : Subsystem  Priority=1  TreatAsAtomicUnit=on  mask{PLCOperandTag=Medium_varistor, PLCBlockType=VariableRead, PLCOperandAccess=Read, PLCPOUType=VariableRead, PLCOperandExpression=xxx_PLC_VAR_Medium_varistor}
      mask prompts: PLCOperandTag "Data Tag:"
      mask init:
      | block = gcb;
      | maskObj = Simulink.Mask.get(block);
      | maskObj.Display = sprintf('disp(''%s'');', PLCOperandTag);
      | slplc.callbacks.initInstruction(block);
      mask Help: web([docroot '/plccoder/ref/variableread' '.html']);
      mask DialogControl PLCBlockTitle Prompt: Data Tag Read
      mask Display: disp('Medium_varistor');
  Variable Read5 : Subsystem  Priority=6  TreatAsAtomicUnit=on  mask{PLCOperandTag=Light_sens, PLCBlockType=VariableRead, PLCOperandAccess=Read, PLCPOUType=VariableRead, PLCOperandExpression=xxx_PLC_VAR_Light_sens}
      mask prompts: PLCOperandTag "Data Tag:"
      mask init:
      | block = gcb;
      | maskObj = Simulink.Mask.get(block);
      | maskObj.Display = sprintf('disp(''%s'');', PLCOperandTag);
      | slplc.callbacks.initInstruction(block);
      mask Help: web([docroot '/plccoder/ref/variableread' '.html']);
      mask DialogControl PLCBlockTitle Prompt: Data Tag Read
      mask Display: disp('Light_sens');
  Variable Read6 : Subsystem  Priority=1  TreatAsAtomicUnit=on  mask{PLCOperandTag=Light_sens, PLCBlockType=VariableRead, PLCOperandAccess=Read, PLCPOUType=VariableRead, PLCOperandExpression=xxx_PLC_VAR_Light_sens}
      mask prompts: PLCOperandTag "Data Tag:"
      mask init:
      | block = gcb;
      | maskObj = Simulink.Mask.get(block);
      | maskObj.Display = sprintf('disp(''%s'');', PLCOperandTag);
      | slplc.callbacks.initInstruction(block);
      mask Help: web([docroot '/plccoder/ref/variableread' '.html']);
      mask DialogControl PLCBlockTitle Prompt: Data Tag Read
      mask Display: disp('Light_sens');
  XIC1 : Subsystem  Priority=3  TreatAsAtomicUnit=on  mask{PLCOperandTag=Varistor, PLCBlockType=XIC, PLCPOUType=Contact, PLCOperandExpression=xxx_PLC_VAR_Varistor}
      mask prompts: PLCOperandTag "Operand Tag:"
      mask init:
      | slplc.callbacks.initInstruction(gcb);
      settings: AttributesFormatString=%<PLCOperandTag>
      mask Help: web([docroot '/plccoder/ref/xic' '.html']);
      mask DialogControl PLCBlockTitle Prompt: Examine If Closed (XIC)
  XIC2 : Subsystem  Priority=2  TreatAsAtomicUnit=on  mask{PLCOperandTag=System_dead, PLCBlockType=XIC, PLCPOUType=Contact, PLCOperandExpression=xxx_PLC_VAR_System_dead}
      mask prompts: PLCOperandTag "Operand Tag:"
      mask init:
      | slplc.callbacks.initInstruction(gcb);
      settings: AttributesFormatString=%<PLCOperandTag>
      mask Help: web([docroot '/plccoder/ref/xic' '.html']);
      mask DialogControl PLCBlockTitle Prompt: Examine If Closed (XIC)
  XIC3 : Subsystem  Priority=3  TreatAsAtomicUnit=on  mask{PLCOperandTag=Light_Low, PLCBlockType=XIC, PLCPOUType=Contact, PLCOperandExpression=xxx_PLC_VAR_Light_Low}
      mask prompts: PLCOperandTag "Operand Tag:"
      mask init:
      | slplc.callbacks.initInstruction(gcb);
      settings: AttributesFormatString=%<PLCOperandTag>
      mask Help: web([docroot '/plccoder/ref/xic' '.html']);
      mask DialogControl PLCBlockTitle Prompt: Examine If Closed (XIC)
  XIC4 : Subsystem  Priority=3  TreatAsAtomicUnit=on  mask{PLCOperandTag=Varistor_low, PLCBlockType=XIC, PLCPOUType=Contact, PLCOperandExpression=xxx_PLC_VAR_Varistor_low}
      mask prompts: PLCOperandTag "Operand Tag:"
      mask init:
      | slplc.callbacks.initInstruction(gcb);
      settings: AttributesFormatString=%<PLCOperandTag>
      mask Help: web([docroot '/plccoder/ref/xic' '.html']);
      mask DialogControl PLCBlockTitle Prompt: Examine If Closed (XIC)
  XIC5 : Subsystem  Priority=3  TreatAsAtomicUnit=on  mask{PLCOperandTag=Varistor_high, PLCBlockType=XIC, PLCPOUType=Contact, PLCOperandExpression=xxx_PLC_VAR_Varistor_high}
      mask prompts: PLCOperandTag "Operand Tag:"
      mask init:
      | slplc.callbacks.initInstruction(gcb);
      settings: AttributesFormatString=%<PLCOperandTag>
      mask Help: web([docroot '/plccoder/ref/xic' '.html']);
      mask DialogControl PLCBlockTitle Prompt: Examine If Closed (XIC)
  XIO : Subsystem  Priority=5  TreatAsAtomicUnit=on  mask{PLCOperandExpression=xxx_PLC_VAR_System_dead, PLCOperandTag=System_dead, PLCBlockType=XIO, PLCPOUType=Contact}
      mask prompts: PLCOperandTag "Operand Tag:"
      mask init:
      | slplc.callbacks.initInstruction(gcb);
      settings: AttributesFormatString=%<PLCOperandTag>
      mask Help: web([docroot '/plccoder/ref/xio' '.html']);
      mask DialogControl PLCBlockTitle Prompt: Examine If Open (XIO)
  XIO1 : Subsystem  Priority=1  TreatAsAtomicUnit=on  mask{PLCOperandExpression=xxx_PLC_VAR_System_dead, PLCOperandTag=System_dead, PLCBlockType=XIO, PLCPOUType=Contact}
      mask prompts: PLCOperandTag "Operand Tag:"
      mask init:
      | slplc.callbacks.initInstruction(gcb);
      settings: AttributesFormatString=%<PLCOperandTag>
      mask Help: web([docroot '/plccoder/ref/xio' '.html']);
      mask DialogControl PLCBlockTitle Prompt: Examine If Open (XIO)
  XIO2 : Subsystem  Priority=1  TreatAsAtomicUnit=on  mask{PLCOperandExpression=xxx_PLC_VAR_System_dead, PLCOperandTag=System_dead, PLCBlockType=XIO, PLCPOUType=Contact}
      mask prompts: PLCOperandTag "Operand Tag:"
      mask init:
      | slplc.callbacks.initInstruction(gcb);
      settings: AttributesFormatString=%<PLCOperandTag>
      mask Help: web([docroot '/plccoder/ref/xio' '.html']);
      mask DialogControl PLCBlockTitle Prompt: Examine If Open (XIO)
  XIO3 : Subsystem  Priority=1  TreatAsAtomicUnit=on  mask{PLCOperandExpression=xxx_PLC_VAR_Light_Low, PLCOperandTag=Light_Low, PLCBlockType=XIO, PLCPOUType=Contact}
      mask prompts: PLCOperandTag "Operand Tag:"
      mask init:
      | slplc.callbacks.initInstruction(gcb);
      settings: AttributesFormatString=%<PLCOperandTag>
      mask Help: web([docroot '/plccoder/ref/xio' '.html']);
      mask DialogControl PLCBlockTitle Prompt: Examine If Open (XIO)
  XIO4 : Subsystem  Priority=1  TreatAsAtomicUnit=on  mask{PLCOperandExpression=xxx_PLC_VAR_Varistor_low, PLCOperandTag=Varistor_low, PLCBlockType=XIO, PLCPOUType=Contact}
      mask prompts: PLCOperandTag "Operand Tag:"
      mask init:
      | slplc.callbacks.initInstruction(gcb);
      settings: AttributesFormatString=%<PLCOperandTag>
      mask Help: web([docroot '/plccoder/ref/xio' '.html']);
      mask DialogControl PLCBlockTitle Prompt: Examine If Open (XIO)
  XIO5 : Subsystem  Priority=1  TreatAsAtomicUnit=on  mask{PLCOperandExpression=xxx_PLC_VAR_Varistor_high, PLCOperandTag=Varistor_high, PLCBlockType=XIO, PLCPOUType=Contact}
      mask prompts: PLCOperandTag "Operand Tag:"
      mask init:
      | slplc.callbacks.initInstruction(gcb);
      settings: AttributesFormatString=%<PLCOperandTag>
      mask Help: web([docroot '/plccoder/ref/xio' '.html']);
      mask DialogControl PLCBlockTitle Prompt: Examine If Open (XIO)
  wires:
  XIO1/1(RungOut) -> XIC1/1(RungIn)
  Power Rail Start/1(PowerOut) -> XIC2/1(RungIn), XIO/1(RungIn), XIO2/1(RungIn), Power Rail Terminal/1(PowerIn), LES2/1(RungIn), NOT1/1(RungIn), XIO1/1(RungIn)
  AND/2(dest) -> OTE/1(RungIn)
  LES/1(RungOut) -> NOT/2(src), OTL1/1(RungIn)
  Variable Read1/1(VarOut) -> LES1/3(srcB)
  OTE/1(RungOut) -> Junction/2(RungIn2)
  OTL1/1(RungOut) -> Junction/1(RungIn1)
  LES1/1(RungOut) -> AND/3(srcB)
  Variable Read/1(VarOut) -> LES/3(srcB)
  NOT/1(RungOut) -> AND/1(RungIn), LES1/1(RungIn)
  NOT/2(dest) -> AND/2(srcA)
  LES4/1(RungOut) -> AND2/3(srcB)
  NOT1/1(RungOut) -> AND1/1(RungIn), LES3/1(RungIn)
  LES2/1(RungOut) -> NOT1/2(src), OTL2/1(RungIn)
  AND1/1(RungOut) -> LES4/1(RungIn), NOT2/1(RungIn)
  OR/2(dest) -> NOT3/2(src)
  NOT3/2(dest) -> OTE3/1(RungIn)
  AND1/2(dest) -> NOT2/2(src), OTE1/1(RungIn)
  LES3/1(RungOut) -> AND1/3(srcB)
  OTE2/1(RungOut) -> OR/3(srcB)
  OTL2/1(RungOut) -> Junction1/1(RungIn1)
  Variable Read3/1(VarOut) -> LES2/3(srcB)
  OTE1/1(RungOut) -> OR/2(srcA)
  Variable Read4/1(VarOut) -> LES4/3(srcB)
  AND2/2(dest) -> OTE2/1(RungIn)
  AND2/1(RungOut) -> OR/1(RungIn)
  Variable Read2/1(VarOut) -> LES3/3(srcB)
  OR/1(RungOut) -> NOT3/1(RungIn)
  OTE3/1(RungOut) -> Junction1/2(RungIn2)
  NOT2/1(RungOut) -> AND2/1(RungIn)
  NOT1/2(dest) -> AND1/2(srcA)
  XIC1/1(RungOut) -> LES2/2(srcA), LES3/2(srcA), LES4/2(srcA)
  NOT2/2(dest) -> AND2/2(srcA)
  Junction1/1(RungOut) -> Rung Terminal2/1(RungIn)
  OTL/1(RungOut) -> Rung Terminal/1(RungIn)
  XIC2/1(RungOut) -> OTL/1(RungIn)
  XIO2/1(RungOut) -> XIO3/1(RungIn), XIC3/1(RungIn)
  XIC3/1(RungOut) -> XIO4/1(RungIn), XIC4/1(RungIn)
  XIC4/1(RungOut) -> OTL3/1(RungIn)
  XIO4/1(RungOut) -> OTU/1(RungIn)
  OTL3/1(RungOut) -> Junction2/1(RungIn1)
  OTU/1(RungOut) -> Junction2/2(RungIn2)
  Junction3/1(RungOut) -> Junction4/2(RungIn2)
  OTL4/1(RungOut) -> Junction3/1(RungIn1)
  XIC5/1(RungOut) -> OTL4/1(RungIn)
  XIO5/1(RungOut) -> OTU1/1(RungIn)
  OTU1/1(RungOut) -> Junction3/2(RungIn2)
  XIO3/1(RungOut) -> XIC5/1(RungIn), XIO5/1(RungIn)
  Junction2/1(RungOut) -> Junction4/1(RungIn1)
  Junction4/1(RungOut) -> Rung Terminal3/1(RungIn)
  Junction/1(RungOut) -> Rung Terminal1/1(RungIn)
  Variable Read5/1(VarOut) -> LES/2(srcA)
  Variable Read6/1(VarOut) -> LES1/2(srcA)
  XIO/1(RungOut) -> NOT/1(RungIn), LES/1(RungIn)
